simulink model "fig93_FAP_fuenteIdeal"  (R2021a)
settings: Solver=ode23tb  StartTime=0.0  StopTime=4/60  RelTol=1e-3  EnableMultiTasking=on
InitFcn:
  | N = 2^11;
  | Ts = 1/(N*60);
libraries: spsCurrentMeasurementLib x9, spsControlledCurrentSourceLib x6, spsGroundLib x4, spsControlledVoltageSourceLib x3, spsVoltageMeasurementLib x3, spsMeanLib x2, spsSequenceAnalyzerLib x1, vrlib x1, spspowerguiLib x1
settings Model: Creator=aj_us  LastModifiedBy=ajust
settings SolverCC: AlgebraicLoopSolver=TrustRegion  SolverResetMethod=Robust
settings DataIOCC: LimitDataPoints=on  ReturnWorkspaceOutputs=off
settings OptimizationCC: LifeSpan=inf
settings DebuggingCC: AllowSymbolicDim=off  SFUnexpectedBacktrackingDiag=warning  SFNoUnconditionalDefaultTransitionDiag=warning  SFExecutionAtInitializationDiag=none  SFMachineParentedDataDiag=warning  ArithmeticOperatorsInVariantConditions=warning
settings ModelReferenceCC: PropagateSignalLabelsOutOfModel=off
settings SFSimCC: SimUseLocalCustomCode=off  CustomCodeUndefinedFunction=UseInterfaceOnly
settings RTWCC: RTWUseLocalCustomCode=off
settings CodeAppCC: StateflowObjectComments=on
settings GRTTargetCC: TargetLangStandard=C89/C90 (ANSI)
settings ConfigComp: CovMetricSettings=dw  CovSaveCumulativeToWorkspaceVar=on  CovSaveSingleToWorkspaceVar=on  CovExternalEMLEnable=off
settings SimscapeCC: SimscapeNormalizeSystem=off

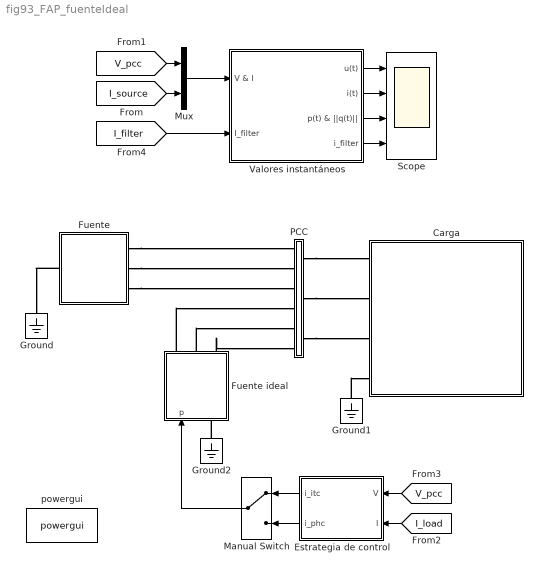
== system fig93_FAP_fuenteIdeal ==
  Carga : Subsystem
      mask Display: plot(0,100,100,100,[0 50 50 0 0],[0 0 100 100 0],[50 75 75 NaN 75 95 95 NaN 71 79],[75 75 53 NaN 75 75 60 NaN 53 53],[50 75 75 NaN 75 95 95 NaN 71 74 76 79],[25 25 50 NaN 25 25 41 NaN 47 50 50 47],[95 91 99 91 99 91 99 95],[60 58 55 52 49 46 43 41],[25 25 15 25 25 NaN 25 35 25 NaN 15 35],[15 30 30 60 85 NaN 30 30 60 NaN 60 60])
  Estrategia de control : Subsystem
  Fuente : Subsystem
      mask Display: plot(-75,-50,75,50,[0,9,18,24,29,30,29,24,18,9,0,-9,-18,-24,-29,-30,-29,-24,-18,-9,0],[30,29,24,18,9,0,-9,-18,-24,-29,-30,-29,-24,-18,-9,0,9,18,24,29,30],[-50 -30],[0 0],[50,30],[0 0],[45 35 40 40 40],[15 15 15 20 10],[0,9,18,24,29,30,29,24,18,9,0,-9,-18,-24,-29,-30,-29,-24,-18,-9,0]./-2.4,[1 2 3 4 5 6 7 8 9 10 11 12 13 14 15 16 17 18 19 20 21].*1.5-15);
  Fuente ideal : Subsystem
      mask Display: plot(-50,-50,50,50,[0,9,18,24,29,30,29,24,18,9,0,-9,-18,-24,-29,-30,-29,-24,-18,-9,0],[30,29,24,18,9,0,-9,-18,-24,-29,-30,-29,-24,-18,-9,0,9,18,24,29,30],[2 2 12 2 -8 2],[-20 5 5 20 5 5]);
  Ground : spsGroundLib/Ground  LConnTagsString=a
  Ground1 : spsGroundLib/Ground  LConnTagsString=a
  Ground2 : spsGroundLib/Ground  LConnTagsString=a
  Manual Switch : ManualSwitch
  Mux : Mux  Inputs=2
  PCC : Subsystem
  Scope : Scope  NumInputPorts=4
  Valores instantáneos : Subsystem
  powergui : spspowerguiLib/powergui  Priority=1  SimulationMode=Discrete  SampleTime=Ts  frequency=60  Iterations=50  frequencyindice=60  Pbase=100e6  ErrMax=1e-4  UnitsV=kV  UnitsW=MW  buscounter=0  FunctionMessages=off  echomessages=off  EnableUseOfTLC=off  CurrentSourceSwitches=off  DisableSnubberDevices=off  DisableRonSwitches=off  DisableVfSwitches=off  DisplayEquations=off  AutomaticDiscreteSolvers=off  SolverType=Tustin/Backward Euler (TBE)  Interpol=off  ExternalGateDelay=off  methode=off  Ts=10  x0status=blocks  SPID=off  SwTol=0  HookPort=off  NonlinearTolerance=1e-4  nMaxIteration=100  ContinueOnMaxIteration=off  RestoreLinks=warning  ResistiveCurrentMeasurement=off  Frange=[0:2:500]  Ylog=off  Xlog=on  ShowGrid=off  save=off  variable=ZData  structure=0  ZoomFFT=off  StartTime=0.0  cycles=1  DisplayStyle=1  fundamental=60  FreqAxis=off  MaxFrequency=1000  frequencyindicesteady=1  RmsSteady=1  display=off
  wires:
  Mux/1 -> Valores instantáneos/1("V & I ")
  [V_pcc] -> Mux/1
  [I_source] -> Mux/2
  Valores instantáneos/1(u(t)) -> Scope/1
  [I_load] -> Estrategia de control/2(I)
  [V_pcc] -> Estrategia de control/1(V)
  Manual Switch/1 -> Fuente ideal/1(p)
  Estrategia de control/1(i_itc) -> Manual Switch/1
  [I_filter] -> Valores instantáneos/2(I_filter)
  Estrategia de control/2(i_phc) -> Manual Switch/2
  Valores instantáneos/2(i(t)) -> Scope/2
  Valores instantáneos/3(p(t) & ||q(t)||) -> Scope/3
  Valores instantáneos/4(i_filter) -> Scope/4
  connections:
  Fuente/LConn1 -- Ground/LConn1
  Ground1/LConn1 -- Carga/LConn4
  PCC/RConn1 -- Carga/LConn1
  PCC/RConn2 -- Carga/LConn2
  PCC/RConn3 -- Carga/LConn3
  Fuente/RConn3 -- PCC/LConn3
  Fuente/RConn2 -- PCC/LConn2
  Fuente/RConn1 -- PCC/LConn1
  Ground2/LConn1 -- Fuente ideal/LConn1
  Fuente ideal/RConn1 -- PCC/LConn4
  Fuente ideal/RConn2 -- PCC/LConn5
  Fuente ideal/RConn3 -- PCC/LConn6

== system fig93_FAP_fuenteIdeal/Carga ==
  Load : Subsystem  mask{Order=[1 3 5 7 9 11 13 15], Amplitude=[62.61 46.84 24.34 6.83 3.924 3.247 1.511 1.661], Phase=[-1.709 1.141 -2.362 0.04757 1.103 -2.969 -1.375 0.3527], Frequency=60, Ts=Ts}
      mask prompts: Order "order [h]:"; Amplitude "Peak amplitude (V):"; Phase "Phase (deg):"; Frequency "Fundamental Frequency (Hz):"; Ts "Sample time:"
      mask Display: plot(0,100,100,100,[0 50 50 0 0],[0 0 100 100 0],[50 75 75 NaN 75 95 95 NaN 71 79],[75 75 53 NaN 75 75 60 NaN 53 53],[50 75 75 NaN 75 95 95 NaN 71 74 76 79],[25 25 50 NaN 25 25 41 NaN 47 50 50 47],[95 91 99 91 99 91 99 95],[60 58 55 52 49 46 43 41],[25 25 15 25 25 NaN 25 35 25 NaN 15 35],[15 30 30 60 85 NaN 30 30 60 NaN 60 60])
  Load1 : Subsystem  mask{Order=[1 3 5 7 9 11 13 15], Amplitude=[32.55 26.33 16.63 7.374 2.235 2.286 1.666 0.886], Phase=[2.459 1.082 -0.3362 -1.899 2.049 -0.5765 -2.491 1.342], Frequency=60, Ts=Ts}
      mask prompts: Order "order [h]:"; Amplitude "Peak amplitude (V):"; Phase "Phase (deg):"; Frequency "Fundamental Frequency (Hz):"; Ts "Sample time:"
      mask Display: plot(0,100,100,100,[0 50 50 0 0],[0 0 100 100 0],[50 75 75 NaN 75 95 95 NaN 71 79],[75 75 53 NaN 75 75 60 NaN 53 53],[50 75 75 NaN 75 95 95 NaN 71 74 76 79],[25 25 50 NaN 25 25 41 NaN 47 50 50 47],[95 91 99 91 99 91 99 95],[60 58 55 52 49 46 43 41],[25 25 15 25 25 NaN 25 35 25 NaN 15 35],[15 30 30 60 85 NaN 30 30 60 NaN 60 60])
  Load2 : Subsystem  mask{Order=[1 3 5 7 9 11 13 15], Amplitude=[42.86 33.65 19.77 7.472 2.54 2.853 1.575 1.138], Phase=[0.3703 1.099 1.775 2.245 1.562 1.364 1.417 0.7694], Frequency=60, Ts=Ts}
      mask prompts: Order "order [h]:"; Amplitude "Peak amplitude (V):"; Phase "Phase (deg):"; Frequency "Fundamental Frequency (Hz):"; Ts "Sample time:"
      mask Display: plot(0,100,100,100,[0 50 50 0 0],[0 0 100 100 0],[50 75 75 NaN 75 95 95 NaN 71 79],[75 75 53 NaN 75 75 60 NaN 53 53],[50 75 75 NaN 75 95 95 NaN 71 74 76 79],[25 25 50 NaN 25 25 41 NaN 47 50 50 47],[95 91 99 91 99 91 99 95],[60 58 55 52 49 46 43 41],[25 25 15 25 25 NaN 25 35 25 NaN 15 35],[15 30 30 60 85 NaN 30 30 60 NaN 60 60])
  A : PMIOPort  Side=Left
  B : PMIOPort  Port=2  Side=Left
  C : PMIOPort  Port=3  Side=Left
  N : PMIOPort  Port=4  Side=Left
  connections:
  Load/LConn1 -- A/RConn1
  Load/LConn2 -- Load1/LConn2 -- N/RConn1 -- Load2/LConn2
  Load1/LConn1 -- B/RConn1
  Load2/LConn1 -- C/RConn1

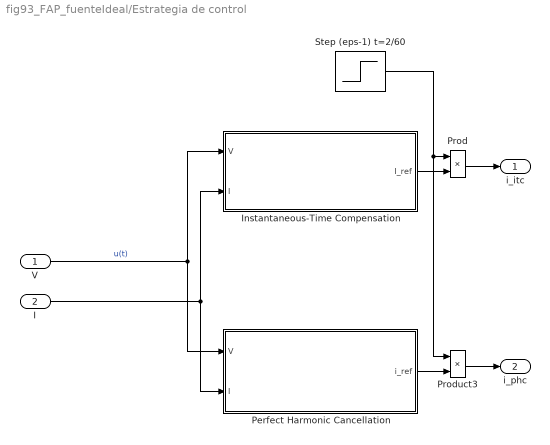
== system fig93_FAP_fuenteIdeal/Estrategia de control ==
  V : Inport
  I : Inport  Port=2
  Instantaneous-Time Compensation : Subsystem
      mask Display:
      | color('green');
      | disp('ITC')
  Perfect Harmonic Cancellation : Subsystem
      mask Display:
      | color('green');
      | disp('PHC')
  Prod : Product
  Product3 : Product
  Step (eps-1) t=2/60 : Step  Time=2/60  Before=eps  SampleTime=0
  i_itc : Outport
  i_phc : Outport  Port=2
  wires:
  V/1 -> Instantaneous-Time Compensation/1(V), Perfect Harmonic Cancellation/1(V)  "u(t)"
  I/1 -> Instantaneous-Time Compensation/2(I), Perfect Harmonic Cancellation/2(I)
  Perfect Harmonic Cancellation/1(i_ref) -> Product3/2
  Product3/1 -> i_phc/1
  Instantaneous-Time Compensation/1(I_ref) -> Prod/2
  Prod/1 -> i_itc/1
  Step (eps-1) t=2/60/1 -> Product3/1, Prod/1

== system fig93_FAP_fuenteIdeal/Fuente ==
  Va : Subsystem  mask{Order=[1], Amplitude=[173.9 ], Phase=[-1.59 ], Frequency=60, Ts=Ts}
      mask prompts: Order "order [h]:"; Amplitude "Peak amplitude (V):"; Phase "Phase (deg):"; Frequency "Fundamental Frequency (Hz):"; Ts "Sample time:"
      mask Display: plot(-50,-50,50,50,[0,9,18,24,29,30,29,24,18,9,0,-9,-18,-24,-29,-30,-29,-24,-18,-9,0],[30,29,24,18,9,0,-9,-18,-24,-29,-30,-29,-24,-18,-9,0,9,18,24,29,30],[-50 -30],[0 0],[50,30],[0 0],[45 35 40 40 40],[15 15 15 20 10],[0,9,18,24,29,30,29,24,18,9,0,-9,-18,-24,-29,-30,-29,-24,-18,-9,0]./-2.4,[1 2 3 4 5 6 7 8 9 10 11 12 13 14 15 16 17 18 19 20 21].*1.5-15);
  Vb : Subsystem  mask{Order=[1], Amplitude=[176.6 ], Phase=[2.613 ], Frequency=60, Ts=Ts}
      mask prompts: Order "order [h]:"; Amplitude "Peak amplitude (V):"; Phase "Phase (deg):"; Frequency "Fundamental Frequency (Hz):"; Ts "Sample time:"
      mask Display: plot(-50,-50,50,50,[0,9,18,24,29,30,29,24,18,9,0,-9,-18,-24,-29,-30,-29,-24,-18,-9,0],[30,29,24,18,9,0,-9,-18,-24,-29,-30,-29,-24,-18,-9,0,9,18,24,29,30],[-50 -30],[0 0],[50,30],[0 0],[45 35 40 40 40],[15 15 15 20 10],[0,9,18,24,29,30,29,24,18,9,0,-9,-18,-24,-29,-30,-29,-24,-18,-9,0]./-2.4,[1 2 3 4 5 6 7 8 9 10 11 12 13 14 15 16 17 18 19 20 21].*1.5-15);
  Vc : Subsystem  mask{Order=[1 ], Amplitude=[175.6 ], Phase=[0.5136 ], Frequency=60, Ts=Ts}
      mask prompts: Order "order [h]:"; Amplitude "Peak amplitude (V):"; Phase "Phase (deg):"; Frequency "Fundamental Frequency (Hz):"; Ts "Sample time:"
      mask Display: plot(-50,-50,50,50,[0,9,18,24,29,30,29,24,18,9,0,-9,-18,-24,-29,-30,-29,-24,-18,-9,0],[30,29,24,18,9,0,-9,-18,-24,-29,-30,-29,-24,-18,-9,0,9,18,24,29,30],[-50 -30],[0 0],[50,30],[0 0],[45 35 40 40 40],[15 15 15 20 10],[0,9,18,24,29,30,29,24,18,9,0,-9,-18,-24,-29,-30,-29,-24,-18,-9,0]./-2.4,[1 2 3 4 5 6 7 8 9 10 11 12 13 14 15 16 17 18 19 20 21].*1.5-15);
  A : PMIOPort  Tag=PMCPort  Side=Right
  B : PMIOPort  Tag=PMCPort  Port=2  Side=Right
  C : PMIOPort  Tag=PMCPort  Port=3  Side=Right
  N : PMIOPort  Tag=PMCPort  Port=4  Side=Left
  connections:
  A/RConn1 -- Va/RConn1
  B/RConn1 -- Vb/RConn1
  C/RConn1 -- Vc/RConn1
  N/RConn1 -- Vc/LConn1 -- Va/LConn1 -- Vb/LConn1

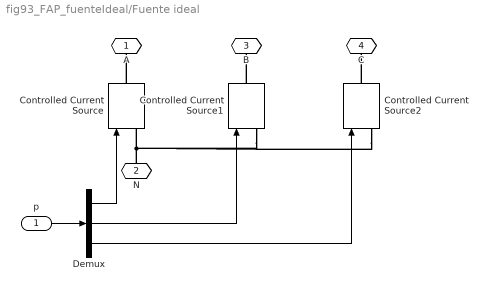
== system fig93_FAP_fuenteIdeal/Fuente ideal ==
  p : Inport
  Controlled Current Source : spsControlledCurrentSourceLib/Controlled Current Source  Initialize=on  Source_Type=AC  Amplitude=0  Phase=0  Frequency=60  Measurements=None
  Controlled Current Source1 : spsControlledCurrentSourceLib/Controlled Current Source  Initialize=on  Source_Type=AC  Amplitude=0  Phase=0  Frequency=60  Measurements=None
  Controlled Current Source2 : spsControlledCurrentSourceLib/Controlled Current Source  Initialize=on  Source_Type=AC  Amplitude=0  Phase=0  Frequency=60  Measurements=None
  Demux : Demux  Outputs=3
  A : PMIOPort  Side=Right
  N : PMIOPort  Port=2  Side=Left
  B : PMIOPort  Port=3  Side=Right
  C : PMIOPort  Port=4  Side=Right
  wires:
  p/1 -> Demux/1
  Demux/1 -> Controlled Current Source/1
  Demux/2 -> Controlled Current Source1/1
  Demux/3 -> Controlled Current Source2/1
  connections:
  N/RConn1 -- Controlled Current Source2/LConn1 -- Controlled Current Source1/LConn1 -- Controlled Current Source/LConn1
  Controlled Current Source/RConn1 -- A/RConn1
  Controlled Current Source1/RConn1 -- B/RConn1
  Controlled Current Source2/RConn1 -- C/RConn1

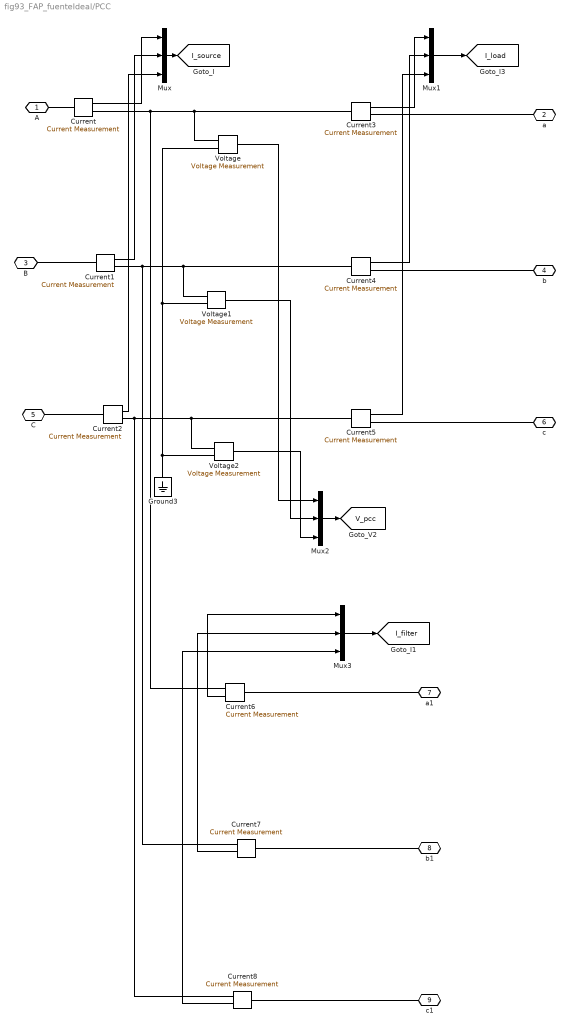
== system fig93_FAP_fuenteIdeal/PCC ==
  Current{,1..8} (9 alike) : spsCurrentMeasurementLib/Current Measurement  PhasorSimulation=off  OutputType=Complex  PSBequivalent=0
  Ground3 : spsGroundLib/Ground  LConnTagsString=a
  Mux{,1..3} (4 alike) : Mux  Inputs=3
  Voltage : spsVoltageMeasurementLib/Voltage Measurement  PhasorSimulation=off  OutputType=Complex  PSBequivalent=0
  Voltage1 : spsVoltageMeasurementLib/Voltage Measurement  PhasorSimulation=off  OutputType=Complex  PSBequivalent=0
  Voltage2 : spsVoltageMeasurementLib/Voltage Measurement  PhasorSimulation=off  OutputType=Complex  PSBequivalent=0
  A : PMIOPort  Side=Left
  a : PMIOPort  Port=2  Side=Right
  B : PMIOPort  Port=3  Side=Left
  b : PMIOPort  Port=4  Side=Right
  C : PMIOPort  Port=5  Side=Left
  c : PMIOPort  Port=6  Side=Right
  a1 : PMIOPort  Port=7  Side=Left
  b1 : PMIOPort  Port=8  Side=Left
  c1 : PMIOPort  Port=9  Side=Left
  tag scope: I_filter=global, I_load=global, I_source=global, V_pcc=global
  wires:
  Voltage1/1 -> Mux2/2
  Voltage2/1 -> Mux2/3
  Mux/1 -> [I_source]
  Current/1 -> Mux/1
  Current1/1 -> Mux/2
  Current2/1 -> Mux/3
  Mux1/1 -> [I_load]
  Current3/1 -> Mux1/1
  Current4/1 -> Mux1/2
  Current5/1 -> Mux1/3
  Mux2/1 -> [V_pcc]
  Voltage/1 -> Mux2/1
  Mux3/1 -> [I_filter]
  Current6/1 -> Mux3/1
  Current7/1 -> Mux3/2
  Current8/1 -> Mux3/3
  connections:
  Voltage/LConn1 -- Current3/LConn1 -- Current6/RConn1 -- Current/RConn1
  Current/LConn1 -- A/RConn1
  Voltage1/LConn1 -- Current4/LConn1 -- Current7/RConn1 -- Current1/RConn1
  Current1/LConn1 -- B/RConn1
  Voltage2/LConn1 -- Current8/RConn1 -- Current2/RConn1 -- Current5/LConn1
  Current2/LConn1 -- C/RConn1
  Voltage1/LConn2 -- Voltage/LConn2 -- Voltage2/LConn2 -- Ground3/LConn1
  Current3/RConn1 -- a/RConn1
  Current5/RConn1 -- c/RConn1
  Current4/RConn1 -- b/RConn1
  Current8/LConn1 -- c1/RConn1
  Current7/LConn1 -- b1/RConn1
  Current6/LConn1 -- a1/RConn1

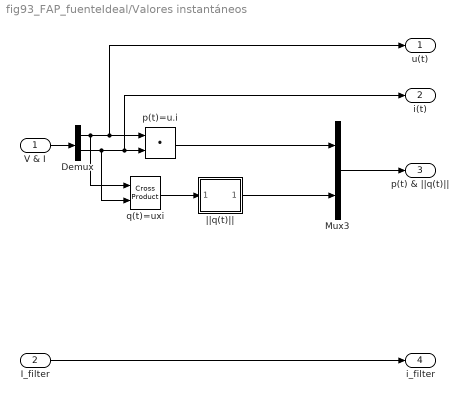
== system fig93_FAP_fuenteIdeal/Valores instantáneos ==
  "V & I " : Inport
  I_filter : Inport  Port=2
  Demux : Demux  Outputs=2
  Mux3 : Mux  Inputs=2
  p(t)=u.i : DotProduct  InputSameDT=on  OutDataTypeStr=Inherit: Inherit via internal rule
  "q(t)=uxi " : vrlib/Utilities/Cross Product
  ||q(t)|| : Subsystem
      mask Display:
      | color blue
      | disp('||u||')
  u(t) : Outport
  i(t) : Outport  Port=2
  p(t) & ||q(t)|| : Outport  Port=3
  i_filter : Outport  Port=4
  wires:
  Demux/2 -> "q(t)=uxi "/2, i(t)/1, p(t)=u.i/2
  "V & I "/1 -> Demux/1
  Mux3/1 -> p(t) & ||q(t)||/1
  Demux/1 -> "q(t)=uxi "/1, u(t)/1, p(t)=u.i/1
  I_filter/1 -> i_filter/1
  "q(t)=uxi "/1 -> ||q(t)||/1(In1)
  p(t)=u.i/1 -> Mux3/1
  ||q(t)||/1(Out1) -> Mux3/2

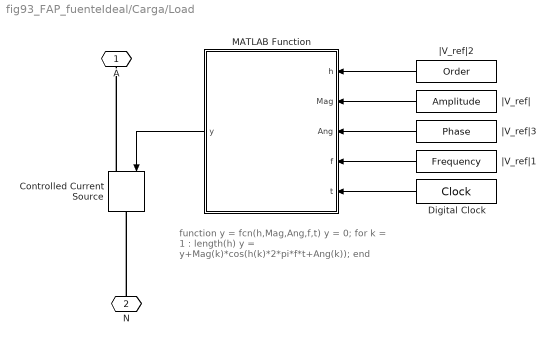
== system fig93_FAP_fuenteIdeal/Carga/Load ==
  note: function y = fcn(h,Mag,Ang,f,t)
      | y = 0;
      | for k = 1 : length(h)
      | y = y+Mag(k)*cos(h(k)*2*pi*f*t+Ang(k));
      | end
  Controlled Current Source : spsControlledCurrentSourceLib/Controlled Current Source  Initialize=on  Source_Type=AC  Amplitude=0  Phase=0  Frequency=60  Measurements=None
  Digital Clock : DigitalClock  SampleTime=Ts
  MATLAB Function : MATLAB Function  TreatAsAtomicUnit=on
  |V_ref| : Constant  Value=Amplitude
  |V_ref|1 : Constant  Value=Frequency
  |V_ref|2 : Constant  Value=Order
  |V_ref|3 : Constant  Value=Phase
  A : PMIOPort  Side=Left
  N : PMIOPort  Port=2  Side=Left
  wires:
  MATLAB Function/1(y) -> Controlled Current Source/1
  |V_ref|3/1 -> MATLAB Function/3(Ang)
  |V_ref|/1 -> MATLAB Function/2(Mag)
  |V_ref|2/1 -> MATLAB Function/1(h)
  |V_ref|1/1 -> MATLAB Function/4(f)
  Digital Clock/1 -> MATLAB Function/5(t)
  connections:
  N/RConn1 -- Controlled Current Source/RConn1
  Controlled Current Source/LConn1 -- A/RConn1

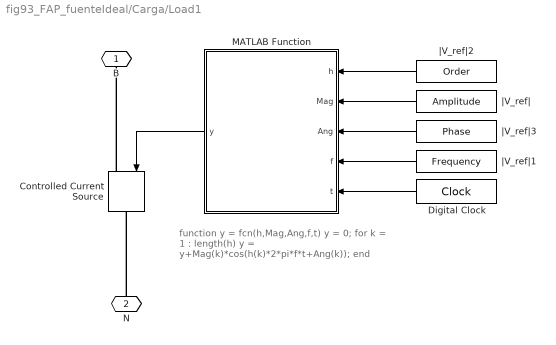
== system fig93_FAP_fuenteIdeal/Carga/Load1 ==
  note: function y = fcn(h,Mag,Ang,f,t)
      | y = 0;
      | for k = 1 : length(h)
      | y = y+Mag(k)*cos(h(k)*2*pi*f*t+Ang(k));
      | end
  Controlled Current Source : spsControlledCurrentSourceLib/Controlled Current Source  Initialize=on  Source_Type=AC  Amplitude=0  Phase=0  Frequency=60  Measurements=None
  Digital Clock : DigitalClock  SampleTime=Ts
  MATLAB Function : MATLAB Function  TreatAsAtomicUnit=on
  |V_ref| : Constant  Value=Amplitude
  |V_ref|1 : Constant  Value=Frequency
  |V_ref|2 : Constant  Value=Order
  |V_ref|3 : Constant  Value=Phase
  B : PMIOPort  Side=Left
  N : PMIOPort  Port=2  Side=Left
  wires:
  MATLAB Function/1(y) -> Controlled Current Source/1
  |V_ref|3/1 -> MATLAB Function/3(Ang)
  |V_ref|/1 -> MATLAB Function/2(Mag)
  |V_ref|2/1 -> MATLAB Function/1(h)
  |V_ref|1/1 -> MATLAB Function/4(f)
  Digital Clock/1 -> MATLAB Function/5(t)
  connections:
  N/RConn1 -- Controlled Current Source/RConn1
  Controlled Current Source/LConn1 -- B/RConn1

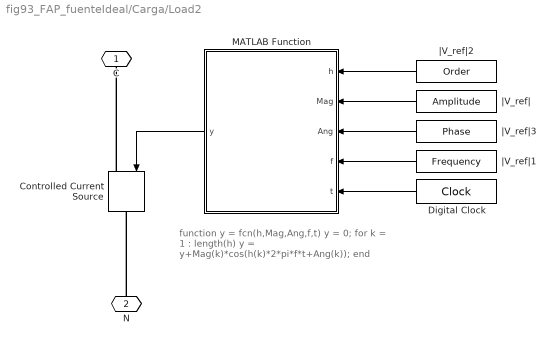
== system fig93_FAP_fuenteIdeal/Carga/Load2 ==
  note: function y = fcn(h,Mag,Ang,f,t)
      | y = 0;
      | for k = 1 : length(h)
      | y = y+Mag(k)*cos(h(k)*2*pi*f*t+Ang(k));
      | end
  Controlled Current Source : spsControlledCurrentSourceLib/Controlled Current Source  Initialize=on  Source_Type=AC  Amplitude=0  Phase=0  Frequency=60  Measurements=None
  Digital Clock : DigitalClock  SampleTime=Ts
  MATLAB Function : MATLAB Function  TreatAsAtomicUnit=on
  |V_ref| : Constant  Value=Amplitude
  |V_ref|1 : Constant  Value=Frequency
  |V_ref|2 : Constant  Value=Order
  |V_ref|3 : Constant  Value=Phase
  C : PMIOPort  Side=Left
  N : PMIOPort  Port=2  Side=Left
  wires:
  MATLAB Function/1(y) -> Controlled Current Source/1
  |V_ref|3/1 -> MATLAB Function/3(Ang)
  |V_ref|/1 -> MATLAB Function/2(Mag)
  |V_ref|2/1 -> MATLAB Function/1(h)
  |V_ref|1/1 -> MATLAB Function/4(f)
  Digital Clock/1 -> MATLAB Function/5(t)
  connections:
  N/RConn1 -- Controlled Current Source/RConn1
  Controlled Current Source/LConn1 -- C/RConn1

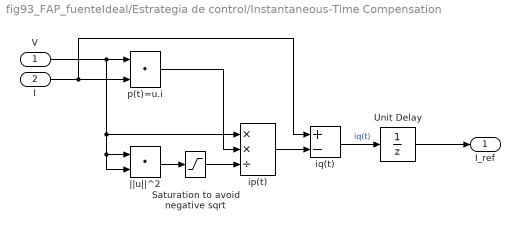
== system fig93_FAP_fuenteIdeal/Estrategia de control/Instantaneous-Time Compensation ==
  V : Inport
  I : Inport  Port=2
  Saturation to avoid negative sqrt : Saturate  UpperLimit=Inf  LowerLimit=eps
  Unit Delay : UnitDelay  SampleTime=-1  HasFrameUpgradeWarning=on
  ip(t) : Product  Inputs=**/
  iq(t) : Sum  Inputs=+-
  p(t)=u.i : DotProduct  InputSameDT=on  OutDataTypeStr=Inherit: Inherit via internal rule
  ||u||^2 : DotProduct  InputSameDT=on  OutDataTypeStr=Inherit: Inherit via internal rule
  I_ref : Outport
  wires:
  I/1 -> p(t)=u.i/2, iq(t)/1
  p(t)=u.i/1 -> ip(t)/2
  V/1 -> ip(t)/1, ||u||^2/2, ||u||^2/1, p(t)=u.i/1
  ||u||^2/1 -> Saturation to avoid negative sqrt/1
  ip(t)/1 -> iq(t)/2
  iq(t)/1 -> Unit Delay/1  "iq(t)"
  Unit Delay/1 -> I_ref/1
  Saturation to avoid negative sqrt/1 -> ip(t)/3

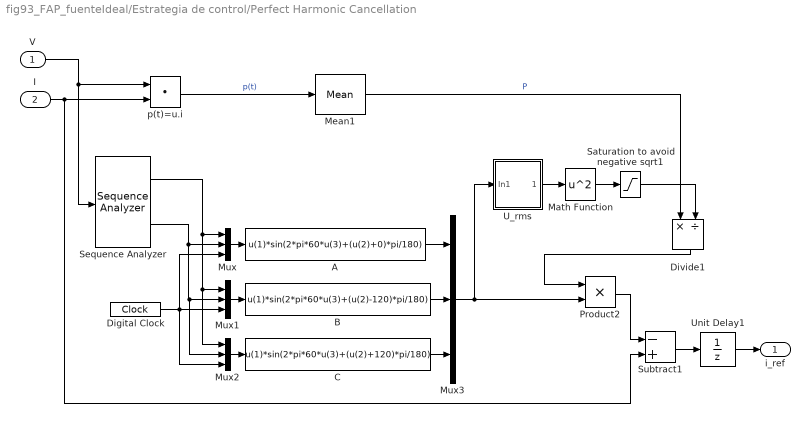
== system fig93_FAP_fuenteIdeal/Estrategia de control/Perfect Harmonic Cancellation ==
  V : Inport
  I : Inport  Port=2
  A : Fcn  Expr=u(1)*sin(2*pi*60*u(3)+(u(2)+0)*pi/180)
  B : Fcn  Expr=u(1)*sin(2*pi*60*u(3)+(u(2)-120)*pi/180)
  C : Fcn  Expr=u(1)*sin(2*pi*60*u(3)+(u(2)+120)*pi/180)
  Digital Clock : DigitalClock  SampleTime=Ts
  Divide1 : Product  Inputs=*/
  Math Function : Math  Operator=square  SignedPower=on  SaturateOnIntegerOverflow=on
  Mean1 : spsMeanLib/Mean  Freq=60  Vinit=0  Ts=Ts
  Mux{,1..3} (4 alike) : Mux  Inputs=3
  Product2 : Product
  Saturation to avoid negative sqrt1 : Saturate  UpperLimit=Inf  LowerLimit=eps
  Sequence Analyzer : spsSequenceAnalyzerLib/Sequence Analyzer  Freq=60  n=1  seq=Positive  InInit=[120, 0]  Ts=Ts
      settings: SourceProductBaseCode=PS
  Subtract1 : Sum  Inputs=-+
  U_rms : Subsystem
      mask Display:
      | color blue
      | disp('RMS_3')
  Unit Delay1 : UnitDelay  SampleTime=-1  HasFrameUpgradeWarning=on
  p(t)=u.i : DotProduct  InputSameDT=on  OutDataTypeStr=Inherit: Inherit via internal rule
  i_ref : Outport
  wires:
  Product2/1 -> Subtract1/1
  Divide1/1 -> Product2/1
  A/1 -> Mux3/1
  Subtract1/1 -> Unit Delay1/1
  I/1 -> p(t)=u.i/2, Subtract1/2
  V/1 -> p(t)=u.i/1, Sequence Analyzer/1
  Unit Delay1/1 -> i_ref/1
  Mean1/1 -> Divide1/1  "P"
  p(t)=u.i/1 -> Mean1/1  "p(t)"
  Mux/1 -> A/1
  Mux1/1 -> B/1
  Mux2/1 -> C/1
  Digital Clock/1 -> Mux1/3, Mux2/3, Mux/3
  Sequence Analyzer/1 -> Mux1/1, Mux2/1, Mux/1
  Sequence Analyzer/2 -> Mux2/2, Mux1/2, Mux/2
  U_rms/1(Out1) -> Math Function/1
  Mux3/1 -> Product2/2, U_rms/1(In1)
  B/1 -> Mux3/2
  C/1 -> Mux3/3
  Math Function/1 -> Saturation to avoid negative sqrt1/1
  Saturation to avoid negative sqrt1/1 -> Divide1/2

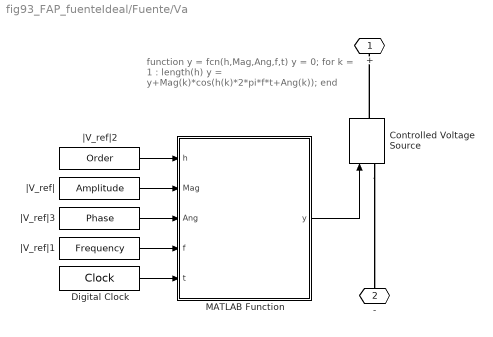
== system fig93_FAP_fuenteIdeal/Fuente/Va ==
  note: function y = fcn(h,Mag,Ang,f,t)
      | y = 0;
      | for k = 1 : length(h)
      | y = y+Mag(k)*cos(h(k)*2*pi*f*t+Ang(k));
      | end
  Controlled Voltage Source : spsControlledVoltageSourceLib/Controlled Voltage Source  Initialize=on  Source_Type=AC  Amplitude=0  Phase=0  Frequency=0  Measurements=None
  Digital Clock : DigitalClock  SampleTime=Ts
  MATLAB Function : MATLAB Function  TreatAsAtomicUnit=on
  |V_ref| : Constant  Value=Amplitude
  |V_ref|1 : Constant  Value=Frequency
  |V_ref|2 : Constant  Value=Order
  |V_ref|3 : Constant  Value=Phase
  + : PMIOPort  Side=Right
  - : PMIOPort  Port=2  Side=Left
  wires:
  MATLAB Function/1(y) -> Controlled Voltage Source/1
  |V_ref|3/1 -> MATLAB Function/3(Ang)
  |V_ref|/1 -> MATLAB Function/2(Mag)
  |V_ref|2/1 -> MATLAB Function/1(h)
  |V_ref|1/1 -> MATLAB Function/4(f)
  Digital Clock/1 -> MATLAB Function/5(t)
  connections:
  Controlled Voltage Source/LConn1 -- -/RConn1
  Controlled Voltage Source/RConn1 -- +/RConn1

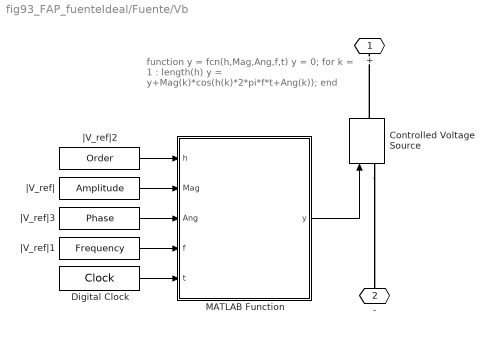
== system fig93_FAP_fuenteIdeal/Fuente/Vb ==
  note: function y = fcn(h,Mag,Ang,f,t)
      | y = 0;
      | for k = 1 : length(h)
      | y = y+Mag(k)*cos(h(k)*2*pi*f*t+Ang(k));
      | end
  Controlled Voltage Source : spsControlledVoltageSourceLib/Controlled Voltage Source  Initialize=on  Source_Type=AC  Amplitude=0  Phase=0  Frequency=0  Measurements=None
  Digital Clock : DigitalClock  SampleTime=Ts
  MATLAB Function : MATLAB Function  TreatAsAtomicUnit=on
  |V_ref| : Constant  Value=Amplitude
  |V_ref|1 : Constant  Value=Frequency
  |V_ref|2 : Constant  Value=Order
  |V_ref|3 : Constant  Value=Phase
  + : PMIOPort  Side=Right
  - : PMIOPort  Port=2  Side=Left
  wires:
  MATLAB Function/1(y) -> Controlled Voltage Source/1
  |V_ref|3/1 -> MATLAB Function/3(Ang)
  |V_ref|/1 -> MATLAB Function/2(Mag)
  |V_ref|2/1 -> MATLAB Function/1(h)
  |V_ref|1/1 -> MATLAB Function/4(f)
  Digital Clock/1 -> MATLAB Function/5(t)
  connections:
  Controlled Voltage Source/LConn1 -- -/RConn1
  Controlled Voltage Source/RConn1 -- +/RConn1

== system fig93_FAP_fuenteIdeal/Fuente/Vc ==
  note: function y = fcn(h,Mag,Ang,f,t)
      | y = 0;
      | for k = 1 : length(h)
      | y = y+Mag(k)*cos(h(k)*2*pi*f*t+Ang(k));
      | end
  Controlled Voltage Source : spsControlledVoltageSourceLib/Controlled Voltage Source  Initialize=on  Source_Type=AC  Amplitude=0  Phase=0  Frequency=0  Measurements=None
  Digital Clock : DigitalClock  SampleTime=Ts
  MATLAB Function : MATLAB Function  TreatAsAtomicUnit=on
  |V_ref| : Constant  Value=Amplitude
  |V_ref|1 : Constant  Value=Frequency
  |V_ref|2 : Constant  Value=Order
  |V_ref|3 : Constant  Value=Phase
  + : PMIOPort  Side=Right
  - : PMIOPort  Port=2  Side=Left
  wires:
  MATLAB Function/1(y) -> Controlled Voltage Source/1
  |V_ref|3/1 -> MATLAB Function/3(Ang)
  |V_ref|/1 -> MATLAB Function/2(Mag)
  |V_ref|2/1 -> MATLAB Function/1(h)
  |V_ref|1/1 -> MATLAB Function/4(f)
  Digital Clock/1 -> MATLAB Function/5(t)
  connections:
  Controlled Voltage Source/LConn1 -- -/RConn1
  Controlled Voltage Source/RConn1 -- +/RConn1

== system fig93_FAP_fuenteIdeal/Valores instantáneos/||q(t)|| ==
  In1 : Inport
  Dot Product : DotProduct  InputSameDT=on  OutDataTypeStr=Inherit: Inherit via internal rule
  Sqrt : Sqrt  SaturateOnIntegerOverflow=on
  Out1 : Outport
  wires:
  In1/1 -> Dot Product/2, Dot Product/1
  Sqrt/1 -> Out1/1
  Dot Product/1 -> Sqrt/1

== system fig93_FAP_fuenteIdeal/Estrategia de control/Perfect Harmonic Cancellation/U_rms ==
  In1 : Inport
  Dot Product : DotProduct  InputSameDT=on  OutDataTypeStr=Inherit: Inherit via internal rule
  Mean : spsMeanLib/Mean  Freq=60  Vinit=0  Ts=Ts
  Saturation to avoid negative sqrt : Saturate  UpperLimit=Inf  LowerLimit=0
  Sqrt : Sqrt  SaturateOnIntegerOverflow=on
  Out1 : Outport
  wires:
  Dot Product/1 -> Mean/1
  In1/1 -> Dot Product/2, Dot Product/1
  Mean/1 -> Saturation to avoid negative sqrt/1
  Saturation to avoid negative sqrt/1 -> Sqrt/1
  Sqrt/1 -> Out1/1

== matlab function fig93_FAP_fuenteIdeal/Carga/Load/MATLAB Function ==
  data: h input; y output; Mag input; Ang input; f input; t input
function y = fcn(h,Mag,Ang,f,t)
y = 0;
for k = 1 : length(h)
    y = y+Mag(k)*cos(h(k)*2*pi*f*t+Ang(k));
end

== matlab function fig93_FAP_fuenteIdeal/Carga/Load1/MATLAB Function ==
  data: h input; y output; Mag input; Ang input; f input; t input
function y = fcn(h,Mag,Ang,f,t)
y = 0;
for k = 1 : length(h)
    y = y+Mag(k)*cos(h(k)*2*pi*f*t+Ang(k));
end

== matlab function fig93_FAP_fuenteIdeal/Fuente/Vb/MATLAB Function ==
  data: h input; y output; Mag input; Ang input; f input; t input
function y = fcn(h,Mag,Ang,f,t)
y = 0;
for k = 1 : length(h)
    y = y+Mag(k)*cos(h(k)*2*pi*f*t+Ang(k));
end

== matlab function fig93_FAP_fuenteIdeal/Fuente/Vc/MATLAB Function ==
  data: h input; y output; Mag input; Ang input; f input; t input
function y = fcn(h,Mag,Ang,f,t)
y = 0;
for k = 1 : length(h)
    y = y+Mag(k)*cos(h(k)*2*pi*f*t+Ang(k));
end

== matlab function fig93_FAP_fuenteIdeal/Fuente/Va/MATLAB Function ==
  data: h input; y output; Mag input; Ang input; f input; t input
function y = fcn(h,Mag,Ang,f,t)
y = 0;
for k = 1 : length(h)
    y = y+Mag(k)*cos(h(k)*2*pi*f*t+Ang(k));
end

== matlab function fig93_FAP_fuenteIdeal/Carga/Load2/MATLAB Function ==
  data: h input; y output; Mag input; Ang input; f input; t input
function y = fcn(h,Mag,Ang,f,t)
y = 0;
for k = 1 : length(h)
    y = y+Mag(k)*cos(h(k)*2*pi*f*t+Ang(k));
end
